simulink model "RT_DAC_UDPInterface"  (R2019b)
settings: Solver=ode5  StartTime=0.0  StopTime=600  RelTol=1e-3  EnableMultiTasking=on
undefined symbols (not defined in the file): Standard_Devices, UDP_Protocol
libraries: simulink x5, sldrtlib x2
settings Model: SimulationMode=external  ExtModeTrigDuration=200000  Creator=Alex  LastModifiedBy=Aleksei
settings DataIOCC: LimitDataPoints=on  SaveFormat=Array  ReturnWorkspaceOutputs=off
settings OptimizationCC: ExpressionDepthLimit=2147483647
settings DebuggingCC: UnderspecifiedInitializationDetection=Classic  MergeDetectMultiDrivingBlocksExec=none  SolverPrmCheckMsg=warning  StateNameClashWarn=warning  SFUnexpectedBacktrackingDiag=warning  SFNoUnconditionalDefaultTransitionDiag=warning  SFExecutionAtInitializationDiag=none  ArithmeticOperatorsInVariantConditions=warning
settings ModelReferenceCC: PropagateSignalLabelsOutOfModel=off
settings SFSimCC: SimUseLocalCustomCode=off  CustomCodeUndefinedFunction=UseInterfaceOnly
settings RTWCC: Description=Simulink Desktop Real-Time  SystemTargetFile=sldrt.tlc  TemplateMakefile=sldrt.tmf  RTWUseLocalCustomCode=off  RTWCompilerOptimization=on
settings CodeAppCC: MaxIdLength=95  StateflowObjectComments=on
settings SimulinkDesktopRealTimeCC: TargetPreCompLibLocation=C:\Program Files\MATLAB\R2019b\toolbox\sldrt\lib\win64  TargetLangStandard=C89/C90 (ANSI)  SupportVariableSizeSignals=off  PreserveStateflowLocalDataDimensions=off
settings ConfigComp: CovMetricSettings=dw  CovHtmlReporting=on  CovSaveCumulativeToWorkspaceVar=on  CovSaveSingleToWorkspaceVar=on  CovExternalEMLEnable=off

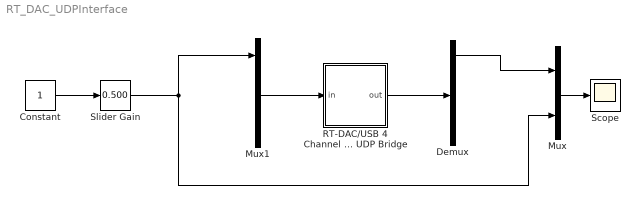
== system RT_DAC_UDPInterface ==
  Constant : Constant
  Demux : Demux
  Mux : Mux  Inputs=2
  Mux1 : Mux
  RT-DAC/USB 4 Channel Analog In/Out via UDP Bridge : Subsystem  mask{Ts=0.05}
      mask prompts: Ts "Sampling interval Ts [s]"
  Scope : Scope
  Slider Gain : simulink/Math Operations/Slider Gain  gain=0.500  low=-1  high=1
  wires:
  Mux/1 -> Scope/1
  Constant/1 -> Slider Gain/1
  Mux1/1 -> RT-DAC/USB 4 Channel Analog In/Out via UDP Bridge/1(in)
  RT-DAC/USB 4 Channel Analog In/Out via UDP Bridge/1(out) -> Demux/1
  Slider Gain/1 -> Mux/2, Mux1/1
  Demux/1 -> Mux/1

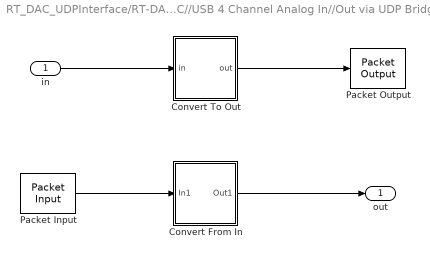
== system RT_DAC_UDPInterface/RT-DAC//USB 4 Channel Analog In//Out via UDP Bridge ==
  in : Inport
  Convert From In : Subsystem
  Convert To Out : Subsystem
  Packet Input : sldrtlib/Packet Input  SampleTime=Ts  MaxMissedTicks=10  ShowMissedTicks=off  YieldWhenWaiting=off  DrvName=Standard_Devices/UDP_Protocol  DrvAddress=6555  DrvOptions=[0 6002 49 50 55 46 48 46 48 46 49 0 0 0 0 0 0 0 0 0 0 0 0 0 0 0 0 0 0 0 0 0 0 0 0 0 0 0 0 0 0 0 0 0 0 0 0 0 0 0 0 0 0 0 0 0 0 0 0 0 0 0 0 0 0 0 0 0 0 0 0 0 0 0 0 0 0 0 0 0 0 0 0 0 0 0 0 0 0 0 0 0 0 0 0 0 0 0 0 0 0 0 0 0 0 0 0 0 0 0 0 0 0 0 0 0 0 0 0 0 0 0 0 0 0 0 0 0 0 0 0 0 0 0 0 0 0 0 0 0 0 0 0 0 0 0 0 0 0 0 0 0 0 0 0 0 0 0 0 0 0 0 0 0 0 0 0 0 0 0 0 0 0 0 0 0 0 0 0 0 0 0 0 0 0 0 0 0 0 0 0 0 0 0 0 0 0 0 0 0 0 0 0 0 0 0 0 0 0 0 0 0 0 0 0 0 0 0 0 0 0 0 0 0 0 0 0 0 0 0 0 0 0 0 0 0 0 0 0 0 0 0 0 0 0 0 0 0 0 0 0 0 0 0 0 0]  PacketSize=8  DataTypes='4*uint16'  ShowReady=off  ShowError=off  PacketID=1  ByteOrder=1  ShowTimestamp=off
      settings: AttributesFormatString=UDP Protocol [6555]  SourceProductName=Simulink Desktop Real-Time
  Packet Output : sldrtlib/Packet Output  SampleTime=Ts  MaxMissedTicks=10  ShowMissedTicks=off  YieldWhenWaiting=off  DrvName=Standard_Devices/UDP_Protocol  DrvAddress=6001  DrvOptions=[0 5666 49 50 55 46 48 46 48 46 49 0 0 0 0 0 0 0 0 0 0 0 0 0 0 0 0 0 0 0 0 0 0 0 0 0 0 0 0 0 0 0 0 0 0 0 0 0 0 0 0 0 0 0 0 0 0 0 0 0 0 0 0 0 0 0 0 0 0 0 0 0 0 0 0 0 0 0 0 0 0 0 0 0 0 0 0 0 0 0 0 0 0 0 0 0 0 0 0 0 0 0 0 0 0 0 0 0 0 0 0 0 0 0 0 0 0 0 0 0 0 0 0 0 0 0 0 0 0 0 0 0 0 0 0 0 0 0 0 0 0 0 0 0 0 0 0 0 0 0 0 0 0 0 0 0 0 0 0 0 0 0 0 0 0 0 0 0 0 0 0 0 0 0 0 0 0 0 0 0 0 0 0 0 0 0 0 0 0 0 0 0 0 0 0 0 0 0 0 0 0 0 0 0 0 0 0 0 0 0 0 0 0 0 0 0 0 0 0 0 0 0 0 0 0 0 0 0 0 0 0 0 0 0 0 0 0 0 0 0 0 0 0 0 0 0 0 0 0 0 0 0 0 0 0 0]  PacketSize=8  DataTypes='4*uint16'  ShowReady=off  ShowError=off  PacketID=1  ByteOrder=1  InitialValue=[]  FinalValue=[]
      settings: AttributesFormatString=UDP Protocol [6001]  SourceProductName=Simulink Desktop Real-Time
  out : Outport
  wires:
  Convert To Out/1(out) -> Packet Output/1
  Packet Input/1 -> Convert From In/1(In1)
  in/1 -> Convert To Out/1(in)
  Convert From In/1(Out1) -> out/1

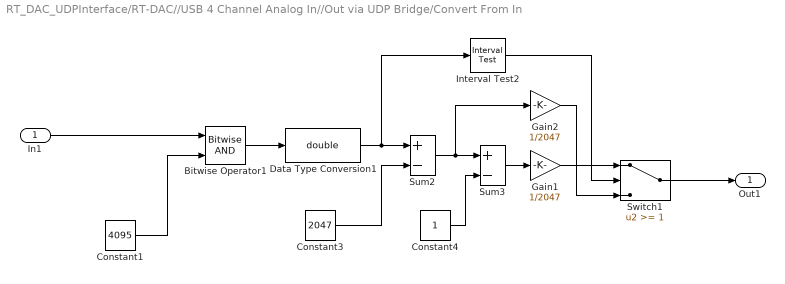
== system RT_DAC_UDPInterface/RT-DAC//USB 4 Channel Analog In//Out via UDP Bridge/Convert From In ==
  In1 : Inport
  Bitwise Operator1 : simulink/Logic and Bit Operations/Bitwise Operator  logicop=AND  UseBitMask=off  NumInputPorts=2  BitMask=bin2dec('11011001')  BitMaskRealWorld=Stored Integer
  Constant1 : Constant  Value=4095  OutDataTypeStr=uint16
  Constant3 : Constant  Value=2047
  Constant4 : Constant
  Data Type Conversion1 : DataTypeConversion  OutDataTypeStr=double
  Gain1 : Gain  Gain=1/2047
  Gain2 : Gain  Gain=1/2047
  Interval Test2 : simulink/Logic and Bit Operations/Interval Test  IntervalClosedRight=on  uplimit=4095  IntervalClosedLeft=on  lowlimit=2048  OutDataTypeStr=uint8
  Sum2 : Sum  Inputs=+-
  Sum3 : Sum  Inputs=+-
  Switch1 : Switch  Threshold=1
  Out1 : Outport
  wires:
  Constant4/1 -> Sum3/2
  Sum3/1 -> Gain1/1
  Interval Test2/1 -> Switch1/2
  Data Type Conversion1/1 -> Interval Test2/1, Sum2/1
  Gain2/1 -> Switch1/3
  Switch1/1 -> Out1/1
  Bitwise Operator1/1 -> Data Type Conversion1/1
  Constant3/1 -> Sum2/2
  Sum2/1 -> Gain2/1, Sum3/1
  Gain1/1 -> Switch1/1
  Constant1/1 -> Bitwise Operator1/2
  In1/1 -> Bitwise Operator1/1

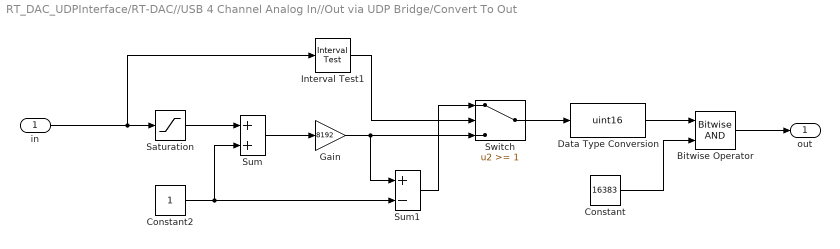
== system RT_DAC_UDPInterface/RT-DAC//USB 4 Channel Analog In//Out via UDP Bridge/Convert To Out ==
  in : Inport
  Bitwise Operator : simulink/Logic and Bit Operations/Bitwise Operator  logicop=AND  UseBitMask=off  NumInputPorts=2  BitMask=bin2dec('11011001')  BitMaskRealWorld=Stored Integer
  Constant : Constant  Value=16383  OutDataTypeStr=uint16
  Constant2 : Constant
  Data Type Conversion : DataTypeConversion  OutDataTypeStr=uint16
  Gain : Gain  Gain=8192
  Interval Test1 : simulink/Logic and Bit Operations/Interval Test  IntervalClosedRight=on  uplimit=1  IntervalClosedLeft=on  lowlimit=0  OutDataTypeStr=uint8
  Saturation : Saturate  UpperLimit=1  LowerLimit=-1
  Sum : Sum
  Sum1 : Sum  Inputs=+-
  Switch : Switch  Threshold=1
  out : Outport
  wires:
  Switch/1 -> Data Type Conversion/1
  Constant2/1 -> Sum1/2, Sum/2
  Sum/1 -> Gain/1
  Data Type Conversion/1 -> Bitwise Operator/1
  Saturation/1 -> Sum/1
  in/1 -> Interval Test1/1, Saturation/1
  Interval Test1/1 -> Switch/2
  Sum1/1 -> Switch/1
  Gain/1 -> Switch/3, Sum1/1
  Constant/1 -> Bitwise Operator/2
  Bitwise Operator/1 -> out/1
